simulink model "Landing_VV"  (R2018b)
settings: Solver=ode4  StartTime=0.0  StopTime=simTime  FixedStep=dt  RelTol=1e-3
InitFcn:
  | SimulationInitialization
StopFcn:
  | SimulationEnd
values from neighbouring files (symbols this model uses):
  Alt = 1000 + TerrainHeight    [SimulationStateConfig.m]
  C = GeneticOpt.C    [SimulationCostFunction.m]
  CartRange_m = MaxAftCartLocX_m - MaxFwdCartLocX_m    (= 1.8505)    [SimulationWSMConfig.m]
  DP_init = 0.5*1.225*V_init^2    [SimulationControlConfig16P.m]    (also in SimulationControlConfig16P_F0.m; SimulationControlConfig16P_F2.m; SimulationControlConfig16P_LEGACY.m; SimulationControlConfigTAILLESS.m)
  dt = DLLSim.dt    [SimulationTimeStep.m]    (also in SimulationTrim.m = 0.02)
  ElevatorMax = 25    [SimulationControlConfig16P.m]    (also in SimulationControlConfig16P_F0.m; SimulationControlConfig16P_F2.m; SimulationControlConfig16P_LEGACY.m; SimulationControlConfigTAILLESS.m)
  EngineLhFuelCut = 0    [SimulationAircraftConfig.m]
  EngineRhFuelCut = 0    [SimulationAircraftConfig.m]
  ftvStaticPositionError = 1/1.18    (= 0.847457627119)    [SimulationSensorConfig16P.m]    (also in SimulationSensorConfig16P_LEGACY.m; SimulationSensorConfigTAILLESS7P.m = 1; SimulationSensorConfigUTAIL7P.m = 1)
  g = 9.81    [SimulationStateConfig.m]
  GustSpd_Kts = testPlans(testIndx).gustSpd    [SimulationStateConfig.m]
  GustTriggerVal = testPlans(testIndx).gustTriggerVal    [SimulationStateConfig.m]
  m = 13.1784    [InertiaEstimatorBWB.m]    (also in SimulationControlConfig16P.m = MassBWB; SimulationControlConfig16P_F0.m = MassBWB; SimulationControlConfig16P_F2.m = MassBWB; SimulationControlConfig16P_LEGACY.m = MassBWB)
  MaxAftCartLocX_m = 2.5327    [SimulationWSMConfig.m]
  MaxFwdCartLocX_m = 0.6822    [SimulationWSMConfig.m]
  nMax_User = 2.6    [SimulationControlConfig16P.m]    (also in SimulationControlConfig16P_F0.m; SimulationControlConfig16P_F2.m; SimulationControlConfig16P_LEGACY.m; SimulationControlConfigTAILLESS.m = 2.5)
  nMin_User = -1.3    [SimulationControlConfig16P.m]    (also in SimulationControlConfig16P_F0.m; SimulationControlConfig16P_F2.m; SimulationControlConfig16P_LEGACY.m; SimulationControlConfigTAILLESS.m = -1)
  SimObj = CompiledSimulink(DLL_Name)    [SimulationTrim.m]
  taxiTrackOffset = testPlans(testIndx).rolloutTrackOffset    [SimulationControlConfig16P.m]    (also in SimulationControlConfig16P_F0.m; SimulationControlConfig16P_F2.m; SimulationControlConfig16P_LEGACY.m; SimulationControlConfigTAILLESS.m)
  V_init = Speed*0.5144    [SimulationControlConfig16P.m]    (also in SimulationControlConfig16P_F0.m; SimulationControlConfig16P_F2.m; SimulationControlConfig16P_LEGACY.m; SimulationControlConfigTAILLESS.m)
  WindDir_Deg = testPlans(testIndx).winds(3)    [SimulationStateConfig.m]
  WindSpd_Kts = testPlans(testIndx).winds(1)    [SimulationStateConfig.m]
  WindVertSpd_Kts = 0    [SimulationStateConfig.m]
  WOWarmed = 1    [SimulationControlConfig16P.m]    (also in SimulationControlConfig16P_F0.m; SimulationControlConfig16P_F2.m; SimulationControlConfig16P_LEGACY.m; SimulationControlConfigTAILLESS.m)
undefined symbols (not defined in the file or in its folder): DiscIntNeverNeededParam, DLLSim, DLLSimStep, sigbuilder_block, Trim_piccoloInCmd, Trim_REFSI_FD_IN_nmodeCgShifterCmd_Flag, Trim_REFSI_FD_IN_nmodeCgShifterCmd_Ft, Trim_REFSI_FD_IN_nmodeCgShifterNRCActive, WSMCart
libraries: Lib_Piccolo x16, simulink x10, aerolibatmos2 x2, Lib_HStab x1
(part 3 of 3)

== system Landing_VV/A//C Dynamics Full Interface/DLLSimulation/Vector to Bus v16_/Vector to Bus 7P - v16 ==
  In1 : Inport
  BusCreator : BusCreator  Inputs=151
  Demux : Demux  Outputs=151
  Out1 : Outport
  wires:
  In1/1 -> Demux/1
  BusCreator/1 -> Out1/1
  Demux/1 -> BusCreator/1  "PresAltFt"
  Demux/2 -> BusCreator/2  "AlphaDeg"
  Demux/3 -> BusCreator/3  "BetaDeg"
  Demux/4 -> BusCreator/4  "GammaDeg"
  Demux/5 -> BusCreator/5  "CASKts"
  Demux/6 -> BusCreator/6  "PDps"
  Demux/7 -> BusCreator/7  "QDps"
  Demux/8 -> BusCreator/8  "RDps"
  Demux/9 -> BusCreator/9  "PhiDeg"
  Demux/10 -> BusCreator/10  "ThetaDeg"
  Demux/11 -> BusCreator/11  "PsiDeg"
  Demux/12 -> BusCreator/12  "TASKts"
  Demux/13 -> BusCreator/13  "HeightAGLFt"
  Demux/14 -> BusCreator/14  "XthrustLbs"
  Demux/15 -> BusCreator/15  "GrndContactLMG"
  Demux/16 -> BusCreator/16  "GrndContactNG"
  Demux/17 -> BusCreator/17  "GrndContactRMG"
  Demux/18 -> BusCreator/18  "DynPresPsf"
  Demux/19 -> BusCreator/19  "PAmbPsf"
  Demux/20 -> BusCreator/20  "XposnFt"
  Demux/21 -> BusCreator/21  "YposnFt"
  Demux/22 -> BusCreator/22  "ZposnFt"
  Demux/23 -> BusCreator/23  "NxG"
  Demux/24 -> BusCreator/24  "NyG"
  Demux/25 -> BusCreator/25  "NzG"
  Demux/26 -> BusCreator/26  "VEarthFtps_0"
  Demux/27 -> BusCreator/27  "VEarthFtps_1"
  Demux/28 -> BusCreator/28  "VEarthFtps_2"
  Demux/29 -> BusCreator/29  "LatitudeDeg"
  Demux/30 -> BusCreator/30  "LongitudeDeg"
  Demux/31 -> BusCreator/31  "ZgrndLhLbs"
  Demux/32 -> BusCreator/32  "ZgrndRhLbs"
  Demux/33 -> BusCreator/33  "ZgrndNgLbs"
  Demux/34 -> BusCreator/34  "Time"
  Demux/35 -> BusCreator/35  "WindUFtps"
  Demux/36 -> BusCreator/36  "WindVFtps"
  Demux/37 -> BusCreator/37  "WindWFtps"
  Demux/38 -> BusCreator/38  "AilLwrLhBDriveDeg"
  Demux/39 -> BusCreator/39  "AilUprLhBDriveDeg"
  Demux/40 -> BusCreator/40  "AilLwrRhBDriveDeg"
  Demux/41 -> BusCreator/41  "AilUprRhBDriveDeg"
  Demux/42 -> BusCreator/42  "ElvLhOBBDriveDeg"
  Demux/43 -> BusCreator/43  "ElvLhIBBDriveDeg"
  Demux/44 -> BusCreator/44  "ElvRhOBBDriveDeg"
  Demux/45 -> BusCreator/45  "ElvRhIBBDriveDeg"
  Demux/46 -> BusCreator/46  "RudPylLhBDriveDeg"
  Demux/47 -> BusCreator/47  "RudUTailLhBDriveDeg"
  Demux/48 -> BusCreator/48  "RudWingletLhBDriveDeg"
  Demux/49 -> BusCreator/49  "ElvUTailLhBDriveDeg"
  Demux/50 -> BusCreator/50  "ElvUTailRhBDriveDeg"
  Demux/51 -> BusCreator/51  "RudPylRhBDriveDeg"
  Demux/52 -> BusCreator/52  "RudUTailRhBDriveDeg"
  Demux/53 -> BusCreator/53  "RudWingletRhBDriveDeg"
  Demux/54 -> BusCreator/54  "AftFlapBDriveDeg"
  Demux/55 -> BusCreator/55  "NWBDriveDeg"
  Demux/56 -> BusCreator/56  "XcgPctMAC"
  Demux/57 -> BusCreator/57  "IxxLbsInch2"
  Demux/58 -> BusCreator/58  "IyyLbsInch2"
  Demux/59 -> BusCreator/59  "IzzLbsInch2"
  Demux/60 -> BusCreator/60  "IxzLbsInch2"
  Demux/61 -> BusCreator/61  "REFSI_FD_OUT_PIC_dynPres_Pa"
  Demux/62 -> BusCreator/62  "REFSI_FD_OUT_PIC_TAmb_C"
  Demux/63 -> BusCreator/63  "REFSI_FD_OUT_PIC_PAmb_Pa"
  Demux/64 -> BusCreator/64  "REFSI_FD_OUT_PIC_rollRate_Dps"
  Demux/65 -> BusCreator/65  "REFSI_FD_OUT_PIC_pitchRate_Dps"
  Demux/66 -> BusCreator/66  "REFSI_FD_OUT_PIC_yawRate_Dps"
  Demux/67 -> BusCreator/67  "REFSI_FD_OUT_PIC_accelXDir_Mps2"
  Demux/68 -> BusCreator/68  "REFSI_FD_OUT_PIC_accelYDir_Mps2"
  Demux/69 -> BusCreator/69  "REFSI_FD_OUT_PIC_accelZDir_Mps2"
  Demux/70 -> BusCreator/70  "REFSI_FD_OUT_PIC_GPSUbloxLatitudeDeg"
  Demux/71 -> BusCreator/71  "REFSI_FD_OUT_PIC_GPSUbloxLongitudeDeg"
  Demux/72 -> BusCreator/72  "REFSI_FD_OUT_PIC_GPSUbloxHeight_m"
  Demux/73 -> BusCreator/73  "REFSI_FD_OUT_PIC_vEarthXUblox_Mps"
  Demux/74 -> BusCreator/74  "REFSI_FD_OUT_PIC_vEarthYUblox_Mps"
  Demux/75 -> BusCreator/75  "REFSI_FD_OUT_PIC_vEarthZUblox_Mps"
  Demux/76 -> BusCreator/76  "REFSI_FD_OUT_PIC_GPSNovAftLatitudeDeg"
  Demux/77 -> BusCreator/77  "REFSI_FD_OUT_PIC_GPSNovAftLongitudeDeg"
  Demux/78 -> BusCreator/78  "REFSI_FD_OUT_PIC_GPSNovAftHeight_m"
  Demux/79 -> BusCreator/79  "REFSI_FD_OUT_PIC_vEarthXNovAft_Mps"
  Demux/80 -> BusCreator/80  "REFSI_FD_OUT_PIC_vEarthYNovAft_Mps"
  Demux/81 -> BusCreator/81  "REFSI_FD_OUT_PIC_vEarthZNovAft_Mps"
  Demux/82 -> BusCreator/82  "ismCas_Kt"
  Demux/83 -> BusCreator/83  "ismTas_Kt"
  Demux/84 -> BusCreator/84  "ismPresAlt_Ft"
  Demux/85 -> BusCreator/85  "ismDynPres_Psf"
  Demux/86 -> BusCreator/86  "ismAoa_Deg"
  Demux/87 -> BusCreator/87  "ismAos_Deg"
  Demux/88 -> BusCreator/88  "speedIncrementImuXRaw_Mps"
  Demux/89 -> BusCreator/89  "speedIncrementImuYRaw_Mps"
  Demux/90 -> BusCreator/90  "speedIncrementImuZRaw_Mps"
  Demux/91 -> BusCreator/91  "rollIncrementRaw_Deg"
  Demux/92 -> BusCreator/92  "pitchIncrementRaw_Deg"
  Demux/93 -> BusCreator/93  "yawIncrementRaw_Deg"
  Demux/94 -> BusCreator/94  "latitudeRaw_Rad"
  Demux/95 -> BusCreator/95  "longitudeRaw_Rad"
  Demux/96 -> BusCreator/96  "heightRaw_M"
  Demux/97 -> BusCreator/97  "speedGpsIneNavXRaw_Mps"
  Demux/98 -> BusCreator/98  "speedGpsIneNavYRaw_Mps"
  Demux/99 -> BusCreator/99  "speedGpsIneNavZRaw_Mps"
  Demux/100 -> BusCreator/100  "isGpsMeasurementValid"
  Demux/101 -> BusCreator/101  "gpsDelay_s"
  Demux/102 -> BusCreator/102  "latitudeStandardDeviation_M"
  Demux/103 -> BusCreator/103  "longitudeStandardDeviation_M"
  Demux/104 -> BusCreator/104  "heightStandardDeviation_M"
  Demux/105 -> BusCreator/105  "speedXStandardDeviation_Mps"
  Demux/106 -> BusCreator/106  "speedYStandardDeviation_Mps"
  Demux/107 -> BusCreator/107  "speedZStandardDeviation_Mps"
  Demux/108 -> BusCreator/108  "gpsMode"
  Demux/109 -> BusCreator/109  "latitudePiccolo_Rad"
  Demux/110 -> BusCreator/110  "longitudePiccolo_Rad"
  Demux/111 -> BusCreator/111  "heightPiccolo_M"
  Demux/112 -> BusCreator/112  "speedGpsIneNavXPiccolo_Mps"
  Demux/113 -> BusCreator/113  "speedGpsIneNavYPiccolo_Mps"
  Demux/114 -> BusCreator/114  "speedGpsIneNavZPiccolo_Mps"
  Demux/115 -> BusCreator/115  "rollAttitudePiccolo_Deg"
  Demux/116 -> BusCreator/116  "pitchAttitudePiccolo_Deg"
  Demux/117 -> BusCreator/117  "yawAttitudePiccolo_Deg"
  Demux/118 -> BusCreator/118  "rollRatePiccolo_Dps"
  Demux/119 -> BusCreator/119  "pitchRatePiccolo_Dps"
  Demux/120 -> BusCreator/120  "yawRatePiccolo_Dps"
  Demux/121 -> BusCreator/121  "nxPiccolo"
  Demux/122 -> BusCreator/122  "nyPiccolo"
  Demux/123 -> BusCreator/123  "nzPiccolo"
  Demux/124 -> BusCreator/124  "piccoloDelay_s"
  Demux/125 -> BusCreator/125  "ismTLALh_Deg"
  Demux/126 -> BusCreator/126  "ismTLARh_Deg"
  Demux/127 -> BusCreator/127  "REFSI_AC_OUT_nmodeRudLhWingCmd_Deg"
  Demux/128 -> BusCreator/128  "REFSI_AC_OUT_nmodeAilLhLowerCmd_Deg"
  Demux/129 -> BusCreator/129  "REFSI_AC_OUT_nmodeAilLhUpperCmd_Deg"
  Demux/130 -> BusCreator/130  "REFSI_AC_OUT_nmodeElvLhOutbdCmd_Deg"
  Demux/131 -> BusCreator/131  "REFSI_AC_OUT_nmodeElvLhInbdCmd_Deg"
  Demux/132 -> BusCreator/132  "REFSI_AC_OUT_nmodeRudLhPylonCmd_Deg"
  Demux/133 -> BusCreator/133  "REFSI_AC_OUT_nmodeRudLhUTailCmd_Deg"
  Demux/134 -> BusCreator/134  "REFSI_AC_OUT_nmodeElvLhUTailCmd_Deg"
  Demux/135 -> BusCreator/135  "REFSI_AC_OUT_nmodeAftFlapCmd_Deg"
  Demux/136 -> BusCreator/136  "REFSI_AC_OUT_nmodeElvRhUTailCmd_Deg"
  Demux/137 -> BusCreator/137  "REFSI_AC_OUT_nmodeRudRhUTailCmd_Deg"
  Demux/138 -> BusCreator/138  "REFSI_AC_OUT_nmodeRudRhPylonCmd_Deg"
  Demux/139 -> BusCreator/139  "REFSI_AC_OUT_nmodeElvRhInbdCmd_Deg"
  Demux/140 -> BusCreator/140  "REFSI_AC_OUT_nmodeElvRhOutbdCmd_Deg"
  Demux/141 -> BusCreator/141  "REFSI_AC_OUT_nmodeAilRhUpperCmd_Deg"
  Demux/142 -> BusCreator/142  "REFSI_AC_OUT_nmodeAilRhLowerCmd_Deg"
  Demux/143 -> BusCreator/143  "REFSI_AC_OUT_nmodeRudRhWingCmd_Deg"
  Demux/144 -> BusCreator/144  "VoltageLhEngine"
  Demux/145 -> BusCreator/145  "VoltageRhEngine"
  Demux/146 -> BusCreator/146  "VoltagePWMLhEngine"
  Demux/147 -> BusCreator/147  "VoltagePWMRhEngine"
  Demux/148 -> BusCreator/148  "CurrentLhEngine"
  Demux/149 -> BusCreator/149  "CurrentRhEngine"
  Demux/150 -> BusCreator/150  "ismN1Lh_Pct"
  Demux/151 -> BusCreator/151  "ismN1Rh_Pct"

== system Landing_VV/A//C Dynamics Full Interface/Gust Wind Input/Gust Wind Model/Gust Models ==
  note: 1) Add Subsystem or Model blocks as valid variant choices.
      | 2) You cannot connect blocks at this level. At simulation, connectivity is automatically
      | determined, based on the active variant and port name matching.
  timeIn_s : Inport
  Continuous Sine : Subsystem  VariantControl="GustType == \"SINE\""  mask{gustMag=GustSpd_Kts, f=0.02}
      mask prompts: gustMag "Gust Magnitude [kts]"; f "Frequency [Hz]"
  Full-Cosine Ramp : Subsystem  VariantControl="GustType == \"FULL\""  mask{gustMag=GustSpd_Kts}
      mask prompts: gustMag "Gust Magnitude [kts]"
  Half-Cosine Ramp : Subsystem  VariantControl="GustType == \"HALF\""  mask{gustMag=GustSpd_Kts}
      mask prompts: gustMag "Gust Magnitude [kts]"
  gustSpdOut_kts : Outport

== system Landing_VV/A//C Dynamics Full Interface/Gust Wind Input/Gust Wind Model/Latch ==
  D : Inport
  Enable/!Rst : Inport  Port=2
  AND : Logic  IconShape=distinctive  AllPortsSameDT=off  OutDataTypeStr=boolean
  Constant : Constant
  OR : Logic  Operator=OR  IconShape=distinctive  AllPortsSameDT=off  OutDataTypeStr=boolean
  Switch : Switch  Criteria=u2 > Threshold  Threshold=0.5
  Unit Delay : UnitDelay  SampleTime=-1
  Q_Latched : Outport
  wires:
  Constant/1 -> Switch/1
  Enable/!Rst/1 -> AND/2
  AND/1 -> Switch/2
  OR/1 -> AND/1
  D/1 -> OR/1, Switch/3
  Switch/1 -> Unit Delay/1, Q_Latched/1
  Unit Delay/1 -> OR/2

== system Landing_VV/A//C Dynamics Full Interface/Gust Wind Input/Gust Wind Model/Timer ==
  Run/!Reset : Inport
  Compare To Constant1 : simulink/Logic and Bit Operations/Compare To Constant  relop=>  const=0  OutDataTypeStr=uint8
  Compare To Constant3 : simulink/Logic and Bit Operations/Compare To Constant  relop===  const=0  OutDataTypeStr=boolean
  Discrete-Time Integrator : DiscreteIntegrator  ExternalReset=level  SampleTime=-1  OutDataTypeStr=double  ICPrevOutput=DiscIntNeverNeededParam  ICPrevScaledInput=DiscIntNeverNeededParam
  timeOut_s : Outport
  wires:
  Compare To Constant1/1 -> Discrete-Time Integrator/1
  Discrete-Time Integrator/1 -> timeOut_s/1
  Run/!Reset/1 -> Compare To Constant1/1, Compare To Constant3/1
  Compare To Constant3/1 -> Discrete-Time Integrator/2

== system Landing_VV/A//C Dynamics Full Interface/Simulated Piccolo Commands/16P5/Signal Builder2 ==
  Demux : Demux  Tag=STV Demux
  FromWs : FromWorkspace  Tag=STV FromWs  VariableName=tuvar  SampleTime=0
      SigBuilderData=|
      | common.afterFinalStr = 'Extrapolate'
      | common.sampleTime = 0
      | dataSet.timeRange = [0 50]
      | dataSet.name = 'Group 1'
      | sbobj.Groups.Name = 'Group 1'
      | sbobj.Groups.Signals(1).Name = 'Signal 3'
      | sbobj.Groups.Signals(1).XData = [0 1 1 50]
      | sbobj.Groups.Signals(1).YData = [0 0 -1 -1]
      | sbobj.Groups.Signals(2).Name = 'Signal 1'
      | sbobj.Groups.Signals(2).XData = [0 20 20 30 30 50]
      | sbobj.Groups.Signals(2).YData = [0 0 0.4 0.4 0 0]
      | sbobj.Groups.Signals(3).Name = 'Signal 2'
      | sbobj.Groups.Signals(3).XData = [0 0.5 0.5 50]
      | sbobj.Groups.Signals(3).YData = [1 1 0 0]
      | sbobj.Groups.Signals(4).Name = 'Signal 4'
      | sbobj.Groups.Signals(4).XData = [0 0.1 0.1 50]
      | sbobj.Groups.Signals(4).YData = [1 1 0 0]
      | sbobj.Groups.TimeRange = [0 50]
  Signal 3 : Outport  Tag=STV Outport
  Signal 1 : Outport  Tag=STV Outport  Port=2
  Signal 2 : Outport  Tag=STV Outport  Port=3
  Signal 4 : Outport  Tag=STV Outport  Port=4
  wires:
  Demux/4 -> Signal 4/1
  Demux/3 -> Signal 2/1
  Demux/2 -> Signal 1/1
  Demux/1 -> Signal 3/1
  FromWs/1 -> Demux/1

== system Landing_VV/A//C Dynamics Full Interface/Simulated Piccolo Commands/16P5/Subsystem ==
  In1 : Inport
  Add : Sum  Inputs=++|
  Bus Selector6 : BusSelector  OutputSignals=REFSI_AC_OUT_nmodeRudLhWingCmd_Deg  OutputAsBus=on
  Product : Product
  CLAWS_RudWingletLhCmdDeg : Outport
  wires:
  [CLAWsOn] -> Product/1
  Product/1 -> Add/1
  Bus Selector6/1 -> Product/2
  In1/1 -> Add/2
  [CLAWsCommands] -> Bus Selector6/1
  Add/1 -> CLAWS_RudWingletLhCmdDeg/1  "REFSI_FD_IN_nmodeRudLhWingCmd_Deg"

== system Landing_VV/A//C Dynamics Full Interface/Simulated Piccolo Commands/16P5/Subsystem1 ==
  In1 : Inport
  Add : Sum  Inputs=++|
  Bus Selector6 : BusSelector  OutputSignals=REFSI_AC_OUT_nmodeAilLhLowerCmd_Deg  OutputAsBus=on
  Product : Product
  CLAWS_AilLwrLhCmdDeg : Outport
  wires:
  Add/1 -> CLAWS_AilLwrLhCmdDeg/1  "REFSI_FD_IN_nmodeAilLhLowerCmd_Deg"
  [CLAWsCommands] -> Bus Selector6/1
  In1/1 -> Add/2
  Bus Selector6/1 -> Product/2
  Product/1 -> Add/1
  [CLAWsOn] -> Product/1

== system Landing_VV/A//C Dynamics Full Interface/Simulated Piccolo Commands/16P5/Subsystem10 ==
  In1 : Inport
  Add : Sum  Inputs=++|
  Bus Selector6 : BusSelector  OutputSignals=REFSI_AC_OUT_nmodeRudRhUTailCmd_Deg
  Product : Product
  CLAWS_RudUTailRhCmdDeg : Outport
  wires:
  [CLAWsOn] -> Product/1
  Product/1 -> Add/1
  Bus Selector6/1 -> Product/2  "<REFSI_AC_OUT_nmodeRudRhUTailCmd_Deg>"
  In1/1 -> Add/2
  [CLAWsCommands] -> Bus Selector6/1
  Add/1 -> CLAWS_RudUTailRhCmdDeg/1  "REFSI_FD_IN_nmodeRudRhUTailCmd_Deg"

== system Landing_VV/A//C Dynamics Full Interface/Simulated Piccolo Commands/16P5/Subsystem11 ==
  In1 : Inport
  Add : Sum  Inputs=++|
  Bus Selector6 : BusSelector  OutputSignals=REFSI_AC_OUT_nmodeRudRhPylonCmd_Deg
  Product : Product
  CLAWS_RudPylRhCmdDeg : Outport
  wires:
  Add/1 -> CLAWS_RudPylRhCmdDeg/1  "REFSI_FD_IN_nmodeRudRhPylonCmd_Deg"
  [CLAWsCommands] -> Bus Selector6/1
  In1/1 -> Add/2
  Bus Selector6/1 -> Product/2  "<REFSI_AC_OUT_nmodeRudRhPylonCmd_Deg>"
  Product/1 -> Add/1
  [CLAWsOn] -> Product/1

== system Landing_VV/A//C Dynamics Full Interface/Simulated Piccolo Commands/16P5/Subsystem12 ==
  In1 : Inport
  Add : Sum  Inputs=++|
  Bus Selector6 : BusSelector  OutputSignals=REFSI_AC_OUT_nmodeElvRhInbdCmd_Deg
  Product : Product
  CLAWS_ElvRhIBCmdDeg : Outport
  wires:
  [CLAWsOn] -> Product/1
  Product/1 -> Add/1
  Bus Selector6/1 -> Product/2  "<REFSI_AC_OUT_nmodeElvRhInbdCmd_Deg>"
  In1/1 -> Add/2
  [CLAWsCommands] -> Bus Selector6/1
  Add/1 -> CLAWS_ElvRhIBCmdDeg/1  "REFSI_FD_IN_nmodeElvRhInbdCmd_Deg"

== system Landing_VV/A//C Dynamics Full Interface/Simulated Piccolo Commands/16P5/Subsystem13 ==
  In1 : Inport
  Add : Sum  Inputs=++|
  Bus Selector6 : BusSelector  OutputSignals=REFSI_AC_OUT_nmodeElvRhOutbdCmd_Deg
  Product : Product
  CLAWS_ElvRhOBCmdDeg : Outport
  wires:
  Add/1 -> CLAWS_ElvRhOBCmdDeg/1  "REFSI_FD_IN_nmodeElvRhOutbdCmd_Deg"
  [CLAWsCommands] -> Bus Selector6/1
  In1/1 -> Add/2
  Bus Selector6/1 -> Product/2  "<REFSI_AC_OUT_nmodeElvRhOutbdCmd_Deg>"
  Product/1 -> Add/1
  [CLAWsOn] -> Product/1

== system Landing_VV/A//C Dynamics Full Interface/Simulated Piccolo Commands/16P5/Subsystem14 ==
  In1 : Inport
  Add : Sum  Inputs=++|
  Bus Selector6 : BusSelector  OutputSignals=REFSI_AC_OUT_nmodeAilRhUpperCmd_Deg
  Product : Product
  CLAWS_AilUprRhCmdDeg : Outport
  wires:
  [CLAWsOn] -> Product/1
  Product/1 -> Add/1
  Bus Selector6/1 -> Product/2  "<REFSI_AC_OUT_nmodeAilRhUpperCmd_Deg>"
  In1/1 -> Add/2
  [CLAWsCommands] -> Bus Selector6/1
  Add/1 -> CLAWS_AilUprRhCmdDeg/1  "REFSI_FD_IN_nmodeAilRhUpperCmd_Deg"

== system Landing_VV/A//C Dynamics Full Interface/Simulated Piccolo Commands/16P5/Subsystem15 ==
  In1 : Inport
  Add : Sum  Inputs=++|
  Bus Selector6 : BusSelector  OutputSignals=REFSI_AC_OUT_nmodeAilRhLowerCmd_Deg
  Product : Product
  CLAWS_AilLwrRhCmdDeg : Outport
  wires:
  Add/1 -> CLAWS_AilLwrRhCmdDeg/1  "REFSI_FD_IN_nmodeAilRhLowerCmd_Deg"
  [CLAWsCommands] -> Bus Selector6/1
  In1/1 -> Add/2
  Bus Selector6/1 -> Product/2  "<REFSI_AC_OUT_nmodeAilRhLowerCmd_Deg>"
  Product/1 -> Add/1
  [CLAWsOn] -> Product/1

== system Landing_VV/A//C Dynamics Full Interface/Simulated Piccolo Commands/16P5/Subsystem16 ==
  In1 : Inport
  Add : Sum  Inputs=++|
  Bus Selector6 : BusSelector  OutputSignals=REFSI_AC_OUT_nmodeRudRhWingCmd_Deg
  Product : Product
  CLAWS_RudWingletRhCmdDeg : Outport
  wires:
  [CLAWsOn] -> Product/1
  Product/1 -> Add/1
  Bus Selector6/1 -> Product/2  "<REFSI_AC_OUT_nmodeRudRhWingCmd_Deg>"
  In1/1 -> Add/2
  [CLAWsCommands] -> Bus Selector6/1
  Add/1 -> CLAWS_RudWingletRhCmdDeg/1  "REFSI_FD_IN_nmodeRudRhWingCmd_Deg"

== system Landing_VV/A//C Dynamics Full Interface/Simulated Piccolo Commands/16P5/Subsystem2 ==
  In1 : Inport
  Add : Sum  Inputs=++|
  Bus Selector6 : BusSelector  OutputSignals=REFSI_AC_OUT_nmodeAilLhUpperCmd_Deg  OutputAsBus=on
  Product : Product
  CLAWS_AilUprLhCmdDeg : Outport
  wires:
  [CLAWsOn] -> Product/1
  Product/1 -> Add/1
  Bus Selector6/1 -> Product/2
  In1/1 -> Add/2
  [CLAWsCommands] -> Bus Selector6/1
  Add/1 -> CLAWS_AilUprLhCmdDeg/1  "REFSI_FD_IN_nmodeAilLhUpperCmd_Deg"

== system Landing_VV/A//C Dynamics Full Interface/Simulated Piccolo Commands/16P5/Subsystem3 ==
  In1 : Inport
  Add : Sum  Inputs=++|
  Bus Selector6 : BusSelector  OutputSignals=REFSI_AC_OUT_nmodeElvLhOutbdCmd_Deg  OutputAsBus=on
  Product : Product
  CLAWS_ElvLhOBCmdDeg : Outport
  wires:
  Add/1 -> CLAWS_ElvLhOBCmdDeg/1  "REFSI_FD_IN_nmodeElvLhOutbdCmd_Deg"
  [CLAWsCommands] -> Bus Selector6/1
  In1/1 -> Add/2
  Bus Selector6/1 -> Product/2
  Product/1 -> Add/1
  [CLAWsOn] -> Product/1

== system Landing_VV/A//C Dynamics Full Interface/Simulated Piccolo Commands/16P5/Subsystem4 ==
  In1 : Inport
  Add : Sum  Inputs=++|
  Bus Selector6 : BusSelector  OutputSignals=REFSI_AC_OUT_nmodeElvLhInbdCmd_Deg  OutputAsBus=on
  Product : Product
  CLAWS_ElvLhIBCmdDeg : Outport
  wires:
  [CLAWsOn] -> Product/1
  Product/1 -> Add/1
  Bus Selector6/1 -> Product/2
  In1/1 -> Add/2
  [CLAWsCommands] -> Bus Selector6/1
  Add/1 -> CLAWS_ElvLhIBCmdDeg/1  "REFSI_FD_IN_nmodeElvLhInbdCmd_Deg"

== system Landing_VV/A//C Dynamics Full Interface/Simulated Piccolo Commands/16P5/Subsystem5 ==
  In1 : Inport
  Add : Sum  Inputs=++|
  Bus Selector6 : BusSelector  OutputSignals=REFSI_AC_OUT_nmodeRudLhPylonCmd_Deg
  Product : Product
  CLAWS_RudPylLhCmdDeg : Outport
  wires:
  Add/1 -> CLAWS_RudPylLhCmdDeg/1  "REFSI_FD_IN_nmodeRudLhPylonCmd_Deg"
  [CLAWsCommands] -> Bus Selector6/1
  In1/1 -> Add/2
  Bus Selector6/1 -> Product/2  "<REFSI_AC_OUT_nmodeRudLhPylonCmd_Deg>"
  Product/1 -> Add/1
  [CLAWsOn] -> Product/1

== system Landing_VV/A//C Dynamics Full Interface/Simulated Piccolo Commands/16P5/Subsystem6 ==
  In1 : Inport
  Add : Sum  Inputs=++|
  Bus Selector6 : BusSelector  OutputSignals=REFSI_AC_OUT_nmodeRudLhUTailCmd_Deg
  Product : Product
  CLAWS_RudUTailLhCmdDeg : Outport
  wires:
  [CLAWsOn] -> Product/1
  Product/1 -> Add/1
  Bus Selector6/1 -> Product/2  "<REFSI_AC_OUT_nmodeRudLhUTailCmd_Deg>"
  In1/1 -> Add/2
  [CLAWsCommands] -> Bus Selector6/1
  Add/1 -> CLAWS_RudUTailLhCmdDeg/1  "REFSI_FD_IN_nmodeRudLhUTailCmd_Deg"

== system Landing_VV/A//C Dynamics Full Interface/Simulated Piccolo Commands/16P5/Subsystem7 ==
  In1 : Inport
  Add : Sum  Inputs=++|
  Bus Selector6 : BusSelector  OutputSignals=REFSI_AC_OUT_nmodeElvLhUTailCmd_Deg
  Product : Product
  CLAWS_ElvUTailLhCmdDeg : Outport
  wires:
  Add/1 -> CLAWS_ElvUTailLhCmdDeg/1  "REFSI_FD_IN_nmodeElvLhUTailCmd_Deg"
  [CLAWsCommands] -> Bus Selector6/1
  In1/1 -> Add/2
  Bus Selector6/1 -> Product/2  "<REFSI_AC_OUT_nmodeElvLhUTailCmd_Deg>"
  Product/1 -> Add/1
  [CLAWsOn] -> Product/1

== system Landing_VV/A//C Dynamics Full Interface/Simulated Piccolo Commands/16P5/Subsystem8 ==
  In1 : Inport
  Add : Sum  Inputs=++|
  Bus Selector6 : BusSelector  OutputSignals=REFSI_AC_OUT_nmodeAftFlapCmd_Deg
  Product : Product
  CLAWS_AftFlapCmdDeg : Outport
  wires:
  [CLAWsOn] -> Product/1
  Product/1 -> Add/1
  Bus Selector6/1 -> Product/2  "<REFSI_AC_OUT_nmodeAftFlapCmd_Deg>"
  In1/1 -> Add/2
  [CLAWsCommands] -> Bus Selector6/1
  Add/1 -> CLAWS_AftFlapCmdDeg/1  "REFSI_FD_IN_nmodeAftFlapCmd_Deg"

== system Landing_VV/A//C Dynamics Full Interface/Simulated Piccolo Commands/16P5/Subsystem9 ==
  In1 : Inport
  Add : Sum  Inputs=++|
  Bus Selector6 : BusSelector  OutputSignals=REFSI_AC_OUT_nmodeElvRhUTailCmd_Deg
  Product : Product
  CLAWS_ElvUTailRhCmdDeg : Outport
  wires:
  Add/1 -> CLAWS_ElvUTailRhCmdDeg/1  "REFSI_FD_IN_nmodeElvRhUTailCmd_Deg"
  [CLAWsCommands] -> Bus Selector6/1
  In1/1 -> Add/2
  Bus Selector6/1 -> Product/2  "<REFSI_AC_OUT_nmodeElvRhUTailCmd_Deg>"
  Product/1 -> Add/1
  [CLAWsOn] -> Product/1

== system Landing_VV/A//C Dynamics Full Interface/Simulated Piccolo Commands/7p/Signal Builder2 ==
  Demux : Demux  Tag=STV Demux
  FromWs : FromWorkspace  Tag=STV FromWs  VariableName=tuvar  SampleTime=0
      SigBuilderData=|
      | common.afterFinalStr = 'Extrapolate'
      | common.sampleTime = 0
      | dataSet.timeRange = [0 50]
      | dataSet.name = 'Group 1'
      | sbobj.Groups.Name = 'Group 1'
      | sbobj.Groups.Signals(1).Name = 'Signal 3'
      | sbobj.Groups.Signals(1).XData = [0 1 1 50]
      | sbobj.Groups.Signals(1).YData = [0 0 -1 -1]
      | sbobj.Groups.Signals(2).Name = 'Signal 1'
      | sbobj.Groups.Signals(2).XData = [0 20 20 30 30 50]
      | sbobj.Groups.Signals(2).YData = [0 0 0.4 0.4 0 0]
      | sbobj.Groups.Signals(3).Name = 'Signal 2'
      | sbobj.Groups.Signals(3).XData = [0 0.5 0.5 50]
      | sbobj.Groups.Signals(3).YData = [1 1 0 0]
      | sbobj.Groups.Signals(4).Name = 'Signal 4'
      | sbobj.Groups.Signals(4).XData = [0 0.1 0.1 50]
      | sbobj.Groups.Signals(4).YData = [1 1 0 0]
      | sbobj.Groups.TimeRange = [0 50]
  Signal 3 : Outport  Tag=STV Outport
  Signal 1 : Outport  Tag=STV Outport  Port=2
  Signal 2 : Outport  Tag=STV Outport  Port=3
  Signal 4 : Outport  Tag=STV Outport  Port=4
  wires:
  Demux/4 -> Signal 4/1
  Demux/3 -> Signal 2/1
  Demux/2 -> Signal 1/1
  Demux/1 -> Signal 3/1
  FromWs/1 -> Demux/1

== system Landing_VV/A//C Dynamics Full Interface/Simulated Piccolo Commands/7p/Subsystem ==
  In1 : Inport
  Add : Sum  Inputs=++|
  Bus Selector6 : BusSelector  OutputSignals=REFSI_AC_OUT_nmodeRudLhWingCmd_Deg  OutputAsBus=on
  Product : Product
  CLAWS_RudWingletLhCmdDeg : Outport
  wires:
  [CLAWsOn] -> Product/1
  Product/1 -> Add/1
  Bus Selector6/1 -> Product/2
  In1/1 -> Add/2
  [CLAWsCommands] -> Bus Selector6/1
  Add/1 -> CLAWS_RudWingletLhCmdDeg/1  "REFSI_FD_IN_nmodeRudLhWingCmd_Deg"

== system Landing_VV/A//C Dynamics Full Interface/Simulated Piccolo Commands/7p/Subsystem1 ==
  In1 : Inport
  Add : Sum  Inputs=++|
  Bus Selector6 : BusSelector  OutputSignals=REFSI_AC_OUT_nmodeAilLhLowerCmd_Deg  OutputAsBus=on
  Product : Product
  CLAWS_AilLwrLhCmdDeg : Outport
  wires:
  Add/1 -> CLAWS_AilLwrLhCmdDeg/1  "REFSI_FD_IN_nmodeAilLhLowerCmd_Deg"
  [CLAWsCommands] -> Bus Selector6/1
  In1/1 -> Add/2
  Bus Selector6/1 -> Product/2
  Product/1 -> Add/1
  [CLAWsOn] -> Product/1

== system Landing_VV/A//C Dynamics Full Interface/Simulated Piccolo Commands/7p/Subsystem10 ==
  In1 : Inport
  Add : Sum  Inputs=++|
  Bus Selector6 : BusSelector  OutputSignals=REFSI_AC_OUT_nmodeRudRhUTailCmd_Deg
  Product : Product
  CLAWS_RudUTailRhCmdDeg : Outport
  wires:
  [CLAWsOn] -> Product/1
  Product/1 -> Add/1
  Bus Selector6/1 -> Product/2  "<REFSI_AC_OUT_nmodeRudRhUTailCmd_Deg>"
  In1/1 -> Add/2
  [CLAWsCommands] -> Bus Selector6/1
  Add/1 -> CLAWS_RudUTailRhCmdDeg/1  "REFSI_FD_IN_nmodeRudRhUTailCmd_Deg"

== system Landing_VV/A//C Dynamics Full Interface/Simulated Piccolo Commands/7p/Subsystem11 ==
  In1 : Inport
  Add : Sum  Inputs=++|
  Bus Selector6 : BusSelector  OutputSignals=REFSI_AC_OUT_nmodeRudRhPylonCmd_Deg
  Product : Product
  CLAWS_RudPylRhCmdDeg : Outport
  wires:
  Add/1 -> CLAWS_RudPylRhCmdDeg/1  "REFSI_FD_IN_nmodeRudRhPylonCmd_Deg"
  [CLAWsCommands] -> Bus Selector6/1
  In1/1 -> Add/2
  Bus Selector6/1 -> Product/2  "<REFSI_AC_OUT_nmodeRudRhPylonCmd_Deg>"
  Product/1 -> Add/1
  [CLAWsOn] -> Product/1

== system Landing_VV/A//C Dynamics Full Interface/Simulated Piccolo Commands/7p/Subsystem12 ==
  In1 : Inport
  Add : Sum  Inputs=++|
  Bus Selector6 : BusSelector  OutputSignals=REFSI_AC_OUT_nmodeElvRhInbdCmd_Deg
  Product : Product
  CLAWS_ElvRhIBCmdDeg : Outport
  wires:
  [CLAWsOn] -> Product/1
  Product/1 -> Add/1
  Bus Selector6/1 -> Product/2  "<REFSI_AC_OUT_nmodeElvRhInbdCmd_Deg>"
  In1/1 -> Add/2
  [CLAWsCommands] -> Bus Selector6/1
  Add/1 -> CLAWS_ElvRhIBCmdDeg/1  "REFSI_FD_IN_nmodeElvRhInbdCmd_Deg"

== system Landing_VV/A//C Dynamics Full Interface/Simulated Piccolo Commands/7p/Subsystem13 ==
  In1 : Inport
  Add : Sum  Inputs=++|
  Bus Selector6 : BusSelector  OutputSignals=REFSI_AC_OUT_nmodeElvRhOutbdCmd_Deg
  Product : Product
  CLAWS_ElvRhOBCmdDeg : Outport
  wires:
  Add/1 -> CLAWS_ElvRhOBCmdDeg/1  "REFSI_FD_IN_nmodeElvRhOutbdCmd_Deg"
  [CLAWsCommands] -> Bus Selector6/1
  In1/1 -> Add/2
  Bus Selector6/1 -> Product/2  "<REFSI_AC_OUT_nmodeElvRhOutbdCmd_Deg>"
  Product/1 -> Add/1
  [CLAWsOn] -> Product/1

== system Landing_VV/A//C Dynamics Full Interface/Simulated Piccolo Commands/7p/Subsystem14 ==
  In1 : Inport
  Add : Sum  Inputs=++|
  Bus Selector6 : BusSelector  OutputSignals=REFSI_AC_OUT_nmodeAilRhUpperCmd_Deg
  Product : Product
  CLAWS_AilUprRhCmdDeg : Outport
  wires:
  [CLAWsOn] -> Product/1
  Product/1 -> Add/1
  Bus Selector6/1 -> Product/2  "<REFSI_AC_OUT_nmodeAilRhUpperCmd_Deg>"
  In1/1 -> Add/2
  [CLAWsCommands] -> Bus Selector6/1
  Add/1 -> CLAWS_AilUprRhCmdDeg/1  "REFSI_FD_IN_nmodeAilRhUpperCmd_Deg"

== system Landing_VV/A//C Dynamics Full Interface/Simulated Piccolo Commands/7p/Subsystem15 ==
  In1 : Inport
  Add : Sum  Inputs=++|
  Bus Selector6 : BusSelector  OutputSignals=REFSI_AC_OUT_nmodeAilRhLowerCmd_Deg
  Product : Product
  CLAWS_AilLwrRhCmdDeg : Outport
  wires:
  Add/1 -> CLAWS_AilLwrRhCmdDeg/1  "REFSI_FD_IN_nmodeAilRhLowerCmd_Deg"
  [CLAWsCommands] -> Bus Selector6/1
  In1/1 -> Add/2
  Bus Selector6/1 -> Product/2  "<REFSI_AC_OUT_nmodeAilRhLowerCmd_Deg>"
  Product/1 -> Add/1
  [CLAWsOn] -> Product/1

== system Landing_VV/A//C Dynamics Full Interface/Simulated Piccolo Commands/7p/Subsystem16 ==
  In1 : Inport
  Add : Sum  Inputs=++|
  Bus Selector6 : BusSelector  OutputSignals=REFSI_AC_OUT_nmodeRudRhWingCmd_Deg
  Product : Product
  CLAWS_RudWingletRhCmdDeg : Outport
  wires:
  [CLAWsOn] -> Product/1
  Product/1 -> Add/1
  Bus Selector6/1 -> Product/2  "<REFSI_AC_OUT_nmodeRudRhWingCmd_Deg>"
  In1/1 -> Add/2
  [CLAWsCommands] -> Bus Selector6/1
  Add/1 -> CLAWS_RudWingletRhCmdDeg/1  "REFSI_FD_IN_nmodeRudRhWingCmd_Deg"

== system Landing_VV/A//C Dynamics Full Interface/Simulated Piccolo Commands/7p/Subsystem2 ==
  In1 : Inport
  Add : Sum  Inputs=++|
  Bus Selector6 : BusSelector  OutputSignals=REFSI_AC_OUT_nmodeAilLhUpperCmd_Deg  OutputAsBus=on
  Product : Product
  CLAWS_AilUprLhCmdDeg : Outport
  wires:
  [CLAWsOn] -> Product/1
  Product/1 -> Add/1
  Bus Selector6/1 -> Product/2
  In1/1 -> Add/2
  [CLAWsCommands] -> Bus Selector6/1
  Add/1 -> CLAWS_AilUprLhCmdDeg/1  "REFSI_FD_IN_nmodeAilLhUpperCmd_Deg"

== system Landing_VV/A//C Dynamics Full Interface/Simulated Piccolo Commands/7p/Subsystem3 ==
  In1 : Inport
  Add : Sum  Inputs=++|
  Bus Selector6 : BusSelector  OutputSignals=REFSI_AC_OUT_nmodeElvLhOutbdCmd_Deg  OutputAsBus=on
  Product : Product
  CLAWS_ElvLhOBCmdDeg : Outport
  wires:
  Add/1 -> CLAWS_ElvLhOBCmdDeg/1  "REFSI_FD_IN_nmodeElvLhOutbdCmd_Deg"
  [CLAWsCommands] -> Bus Selector6/1
  In1/1 -> Add/2
  Bus Selector6/1 -> Product/2
  Product/1 -> Add/1
  [CLAWsOn] -> Product/1

== system Landing_VV/A//C Dynamics Full Interface/Simulated Piccolo Commands/7p/Subsystem4 ==
  In1 : Inport
  Add : Sum  Inputs=++|
  Bus Selector6 : BusSelector  OutputSignals=REFSI_AC_OUT_nmodeElvLhInbdCmd_Deg  OutputAsBus=on
  Product : Product
  CLAWS_ElvLhIBCmdDeg : Outport
  wires:
  [CLAWsOn] -> Product/1
  Product/1 -> Add/1
  Bus Selector6/1 -> Product/2
  In1/1 -> Add/2
  [CLAWsCommands] -> Bus Selector6/1
  Add/1 -> CLAWS_ElvLhIBCmdDeg/1  "REFSI_FD_IN_nmodeElvLhInbdCmd_Deg"

== system Landing_VV/A//C Dynamics Full Interface/Simulated Piccolo Commands/7p/Subsystem5 ==
  In1 : Inport
  Add : Sum  Inputs=++|
  Bus Selector6 : BusSelector  OutputSignals=REFSI_AC_OUT_nmodeRudLhPylonCmd_Deg
  Product : Product
  CLAWS_RudPylLhCmdDeg : Outport
  wires:
  Add/1 -> CLAWS_RudPylLhCmdDeg/1  "REFSI_FD_IN_nmodeRudLhPylonCmd_Deg"
  [CLAWsCommands] -> Bus Selector6/1
  In1/1 -> Add/2
  Bus Selector6/1 -> Product/2  "<REFSI_AC_OUT_nmodeRudLhPylonCmd_Deg>"
  Product/1 -> Add/1
  [CLAWsOn] -> Product/1

== system Landing_VV/A//C Dynamics Full Interface/Simulated Piccolo Commands/7p/Subsystem6 ==
  In1 : Inport
  Add : Sum  Inputs=++|
  Bus Selector6 : BusSelector  OutputSignals=REFSI_AC_OUT_nmodeRudLhUTailCmd_Deg
  Product : Product
  CLAWS_RudUTailLhCmdDeg : Outport
  wires:
  [CLAWsOn] -> Product/1
  Product/1 -> Add/1
  Bus Selector6/1 -> Product/2  "<REFSI_AC_OUT_nmodeRudLhUTailCmd_Deg>"
  In1/1 -> Add/2
  [CLAWsCommands] -> Bus Selector6/1
  Add/1 -> CLAWS_RudUTailLhCmdDeg/1  "REFSI_FD_IN_nmodeRudLhUTailCmd_Deg"

== system Landing_VV/A//C Dynamics Full Interface/Simulated Piccolo Commands/7p/Subsystem7 ==
  In1 : Inport
  Add : Sum  Inputs=++|
  Bus Selector6 : BusSelector  OutputSignals=REFSI_AC_OUT_nmodeElvLhUTailCmd_Deg
  Product : Product
  CLAWS_ElvUTailLhCmdDeg : Outport
  wires:
  Add/1 -> CLAWS_ElvUTailLhCmdDeg/1  "REFSI_FD_IN_nmodeElvLhUTailCmd_Deg"
  [CLAWsCommands] -> Bus Selector6/1
  In1/1 -> Add/2
  Bus Selector6/1 -> Product/2  "<REFSI_AC_OUT_nmodeElvLhUTailCmd_Deg>"
  Product/1 -> Add/1
  [CLAWsOn] -> Product/1

== system Landing_VV/A//C Dynamics Full Interface/Simulated Piccolo Commands/7p/Subsystem8 ==
  In1 : Inport
  Add : Sum  Inputs=++|
  Bus Selector6 : BusSelector  OutputSignals=REFSI_AC_OUT_nmodeAftFlapCmd_Deg
  Product : Product
  CLAWS_AftFlapCmdDeg : Outport
  wires:
  [CLAWsOn] -> Product/1
  Product/1 -> Add/1
  Bus Selector6/1 -> Product/2  "<REFSI_AC_OUT_nmodeAftFlapCmd_Deg>"
  In1/1 -> Add/2
  [CLAWsCommands] -> Bus Selector6/1
  Add/1 -> CLAWS_AftFlapCmdDeg/1  "REFSI_FD_IN_nmodeAftFlapCmd_Deg"

== system Landing_VV/A//C Dynamics Full Interface/Simulated Piccolo Commands/7p/Subsystem9 ==
  In1 : Inport
  Add : Sum  Inputs=++|
  Bus Selector6 : BusSelector  OutputSignals=REFSI_AC_OUT_nmodeElvRhUTailCmd_Deg
  Product : Product
  CLAWS_ElvUTailRhCmdDeg : Outport
  wires:
  Add/1 -> CLAWS_ElvUTailRhCmdDeg/1  "REFSI_FD_IN_nmodeElvRhUTailCmd_Deg"
  [CLAWsCommands] -> Bus Selector6/1
  In1/1 -> Add/2
  Bus Selector6/1 -> Product/2  "<REFSI_AC_OUT_nmodeElvRhUTailCmd_Deg>"
  Product/1 -> Add/1
  [CLAWsOn] -> Product/1

== system Landing_VV/A//C Dynamics Full Interface/Gust Wind Input/Gust Wind Model/Gust Models/Continuous Sine ==
  timeIn_s : Inport
  Gain11 : Gain  Gain=(2*pi*f)
  Gain12 : Gain  Gain=gustMag
  Sin : Trigonometry
  gustSpdOut_kts : Outport
  wires:
  Gain12/1 -> gustSpdOut_kts/1  "RefWindSpdKts"
  timeIn_s/1 -> Gain11/1
  Sin/1 -> Gain12/1
  Gain11/1 -> Sin/1

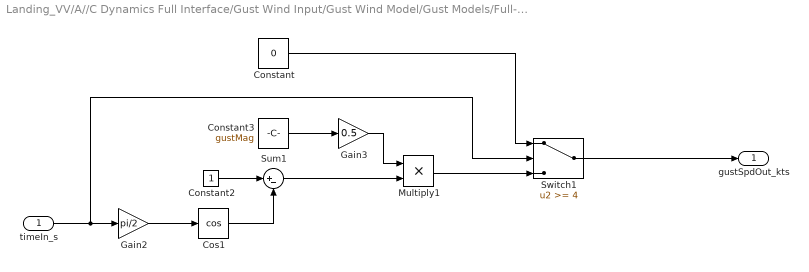
== system Landing_VV/A//C Dynamics Full Interface/Gust Wind Input/Gust Wind Model/Gust Models/Full-Cosine Ramp ==
  timeIn_s : Inport
  Constant : Constant  Value=0
  Constant2 : Constant
  Constant3 : Constant  Value=gustMag
  Cos1 : Trigonometry  Operator=cos
  Gain2 : Gain  Gain=pi/2
  Gain3 : Gain  Gain=0.5
  Multiply1 : Product
  Sum1 : Sum  Inputs=|+-
  Switch1 : Switch  Threshold=4
  gustSpdOut_kts : Outport
  wires:
  Switch1/1 -> gustSpdOut_kts/1
  Constant/1 -> Switch1/1
  Cos1/1 -> Sum1/2
  Gain3/1 -> Multiply1/1
  Constant3/1 -> Gain3/1
  Multiply1/1 -> Switch1/3
  Constant2/1 -> Sum1/1
  Gain2/1 -> Cos1/1
  timeIn_s/1 -> Gain2/1, Switch1/2
  Sum1/1 -> Multiply1/2

== system Landing_VV/A//C Dynamics Full Interface/Gust Wind Input/Gust Wind Model/Gust Models/Half-Cosine Ramp ==
  timeIn_s : Inport
  Constant : Constant
  Constant1 : Constant  Value=gustMag
  Cos : Trigonometry  Operator=cos
  Gain : Gain  Gain=pi/2
  Gain1 : Gain  Gain=0.5
  Multiply : Product
  Sum : Sum  Inputs=|+-
  Switch : Switch  Threshold=2
  gustSpdOut_kts : Outport
  wires:
  Switch/1 -> gustSpdOut_kts/1
  timeIn_s/1 -> Gain/1, Switch/2
  Cos/1 -> Sum/2
  Sum/1 -> Multiply/2
  Gain/1 -> Cos/1
  Constant/1 -> Sum/1
  Multiply/1 -> Switch/3
  Constant1/1 -> Gain1/1, Switch/1
  Gain1/1 -> Multiply/1

== matlab function Landing_VV/A//C Dynamics Full Interface/Raw Sensor Sources Alternate/MATLAB Function ==
  data: u input; y output
function y = fcn(u)
if u > 180
    y = u-360;
else
    y = u;
end
